simulink model "speech_non_uniform"  (Simulink 7.9)
settings: Solver=FixedStepDiscrete  StartTime=0.0  StopTime=10  FixedStep=1/fs  RelTol=1e-3
values from neighbouring files (symbols this model uses):
  A = 87.6    [speech_quant_non_uniform.m]    (also in speech_quant_uniform.m)
  fs = 10*R    (= 10000)    [quant_non_uniform.m]    (also in quant_uniform.m)
  k = 1/4.902/(sqrt(10^(atenuation_dB/10)))    [quant_non_uniform.m]    (also in quant_uniform.m; speech_quant_non_uniform.m = sqrt(10^(atenuation_dB/10)); speech_quant_uniform.m = sqrt(10^(atenuation_dB/10)))
libraries: commsrccod2 x2, dspquant2 x1, dspsrcs4 x1
settings Model: Creator=amoura  LastModifiedBy=amoura_2
settings OptimizationCC: InitFltsAndDblsToZero=on
settings DebuggingCC: SaveWithParameterizedLinksMsg=none  SignalResolutionControl=TryResolveAllWithWarning  FcnCallInpInsideContextMsg=Use local settings  StrictBusMsg=Warning
settings GRTTargetCC: TargetFcnLib=ansi_tfl_tmw.mat  CombineOutputUpdateFcns=off  GRTInterface=on

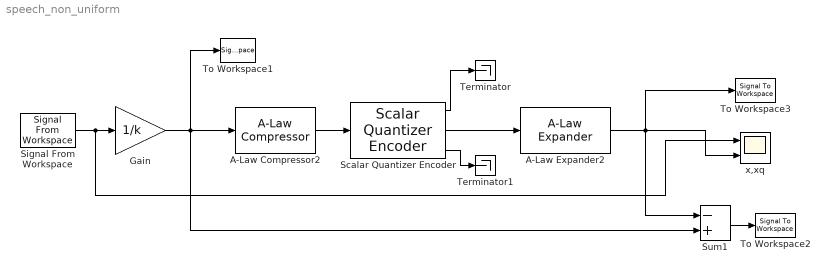
== system speech_non_uniform ==
  A-Law Compressor2 : commsrccod2/A-Law Compressor  A=A  V=1
  A-Law Expander2 : commsrccod2/A-Law Expander  A=A  V=1
  Gain : Gain  Gain=1/k  SaturateOnIntegerOverflow=on  OutDataTypeStr=Inherit: Same as input  ParamDataTypeStr=Inherit: Same as input
  Scalar Quantizer Encoder : dspquant2/Scalar Quantizer Encoder  paramSrc=Specify via dialog  partType=Bounded  BBoundary=boundary  UBoundary=[2:9]  SearchMethod=Linear  tieBreakRule=Choose the lower index  outQU=on  outQError=on  codebook=codebook  outStatus=off  invalidin=Clip  idtype=int32  roundingMode=Floor  overflowMode=off
  Signal From Workspace : dspsrcs4/Signal From Workspace  X=x  Ts=1/fs  nsamps=1  OutputAfterFinalValue=Setting to zero  ignoreOrWarnInputAndFrameLengths=off
  Sum1 : Sum  Inputs=-+  SaturateOnIntegerOverflow=on  InputSameDT=on  OutDataTypeStr=Inherit: Same as first input
  Terminator : Terminator
  Terminator1 : Terminator
  To Workspace1 : SignalToWorkspace  VariableName=xout
  To Workspace2 : SignalToWorkspace  VariableName=eq
  To Workspace3 : SignalToWorkspace  VariableName=xq
  x,xq : Scope  NumInputPorts=2
      settings: TickLabels=on  YMin=-1~-1  YMax=1~1
  wires:
  Signal From Workspace/1 -> Gain/1, x,xq/1
  Scalar Quantizer Encoder/1 -> Terminator/1
  Scalar Quantizer Encoder/3 -> Terminator1/1
  Gain/1 -> To Workspace1/1, Sum1/2, A-Law Compressor2/1
  Sum1/1 -> To Workspace2/1
  Scalar Quantizer Encoder/2 -> A-Law Expander2/1
  A-Law Compressor2/1 -> Scalar Quantizer Encoder/1
  A-Law Expander2/1 -> Sum1/1, x,xq/2, To Workspace3/1
